simulink model "UAVTrimh"  (R2022a)
settings: Solver=ode45  StartTime=0.0  StopTime=50  RelTol=1e-3  EnableMultiTasking=on
values from neighbouring files (symbols this model uses):
  W = 2.5    [Calculos00_OriginalIgnacio.m]    (also in Calculos02_Vnoladetrim.m; Calculos03_TablaTrimados.m; GenerateDataset_v0.m; PI_0_OnlyOneController_V20.m)
  XCG = 0.33    [Calculos00_OriginalIgnacio.m]    (also in Calculos02_Vnoladetrim.m; Calculos03_TablaTrimados.m; GenerateDataset_v0.m; PI_0_OnlyOneController_V20.m)
settings Model: Creator=Ignacio  LastModifiedBy=ignac
settings SolverCC: AlgebraicLoopSolver=TrustRegion
settings DataIOCC: ExternalInput=[0 0.369809473744665 -0.0760167506859634 0.299999999999976]  InitialState=[]  LimitDataPoints=on  SaveFormat=Array  SignalLoggingSaveFormat=ModelDataLogs  ReturnWorkspaceOutputs=off
settings OptimizationCC: DefaultParameterBehavior=Inlined  BufferReuse=off  ExpressionDepthLimit=2147483647  LifeSpan=inf
settings DebuggingCC: UnderspecifiedInitializationDetection=Classic  MergeDetectMultiDrivingBlocksExec=none  FcnCallInpInsideContextMsg=warning  UnconnectedInputMsg=warning  UnconnectedOutputMsg=warning  UnconnectedLineMsg=warning  StateNameClashWarn=warning  InitInArrayFormatMsg=none  SFUnexpectedBacktrackingDiag=warning  SFNoUnconditionalDefaultTransitionDiag=warning  SFExecutionAtInitializationDiag=none  SFMachineParentedDataDiag=warning  ArithmeticOperatorsInVariantConditions=warning
settings HardwareCC: ProdBitPerPointer=32  ProdBitPerSizeT=32  ProdBitPerPtrDiffT=32  ProdLargestAtomicFloat=None  ProdIntDivRoundTo=Undefined  ProdEndianess=Unspecified  ProdWordSize=32  ProdHWDeviceType=32-bit Generic
settings ModelReferenceCC: PropagateSignalLabelsOutOfModel=off
settings SFSimCC: SimUseLocalCustomCode=off  CustomCodeUndefinedFunction=UseInterfaceOnly
settings RTWCC: RTWUseLocalCustomCode=off
settings CodeAppCC: StateflowObjectComments=on
settings GRTTargetCC: TargetLangStandard=C89/C90 (ANSI)
settings ConfigComp: CovMetricSettings=dw  CovSaveCumulativeToWorkspaceVar=on  CovSaveSingleToWorkspaceVar=on  CovExternalEMLEnable=off

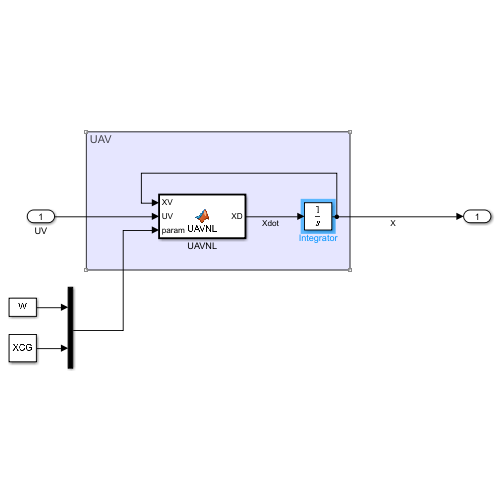
[thumbnail: Simulink's stored preview of the top-level diagram]
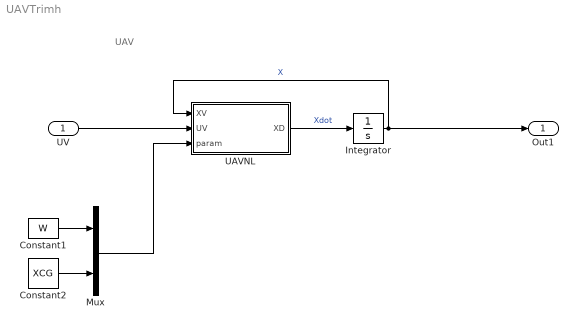
== system UAVTrimh ==
  note: UAV
  UV : Inport  PortDimensions=2
  Constant1 : Constant  Value=W
  Constant2 : Constant  Value=XCG
  Integrator : Integrator  InitialCondition=zeros(1,5)
  Mux : Mux  Inputs=2
  UAVNL : MATLAB Function  TreatAsAtomicUnit=on
  Out1 : Outport
  wires:
  UAVNL/1(XD) -> Integrator/1  "Xdot"
  Integrator/1 -> Out1/1, UAVNL/1(XV)  "X"
  UV/1 -> UAVNL/2(UV)
  Constant1/1 -> Mux/1
  Constant2/1 -> Mux/2
  Mux/1 -> UAVNL/3(param)

== matlab function UAVTrimh/UAVNL ==
  data: XV input; XD output; UV input; param input
function XD = UAVNL(XV,UV,param)

XD=zeros(5,1); % Inicializamos el vector de las derivadas con ceros

% DATOS DE LA AERONAVE

S = 0.4121;               % superficie alar (m^2)
C=0.2192;                  % cuerda media aerodinámica (m)
MASA=2.5;                  % Masa (Kg)
XCGR=0.33;                % posición de referencia del CG
IP=0.156794;                   % Momento de inercia (Kg*m^2)
d=1.225;                      % densidad (Kg/m^3)
G=9.8;                    % gravedad m/s^2
XCG=.33;                  % CG no coincide con el de referencia

% derivadas de estabilidad y control adimensionales

CLalpha0=0.405;    
CLalpha=5.379292;
CLq=11.133615;
CD0=0.0277;
CDalpha=0.14897;
CDalpha2=0.9848;
Cm0=0.0418;     
Cmalpha=-6.0; %1.812981 Más inestable en cabeceo
Cmalphadot=-7.0;
Cmde=-1.552;
Cmq=-18.422237;

% variables de estado


VT=XV(1);	% Velocidad 
ALPHA=XV(2);	% Angulo de ataque
THETA=XV(3);% Angulo de asiento
Q=XV(4);	% Velocidad angular de cabeceo
H=XV(5);

% variables de control

Dt=UV(1);	% Acelerador
De=UV(2);	% Deflexión del timón de profundidad

% parameters

MASA=param(1);
XCG=param(2);

% Density at altitude H
d=density(H);

% Algunos calculos previos

U=VT*cos(ALPHA);	% Componentes de la velocidad en ejes cuerpo
W=VT*sin(ALPHA);	

PDS=0.5*d*(VT^2)*S;	% Presión dinámica*Superficie alar

% Parametros Grupo Motopropulsor

Dh=0.254;   % Diametro de la helice (m)

REVmax=222; % Revoluciones maximas del motor (rev/s)

CT0=0.13805; % Coeficientes de traccion
CTj=-0.2049;
REV=REVmax*Dt; % Motor instantaneo
J=VT/(REV*Dh);  %Coef de velocidad
C_T=CT0+CTj*J;          %Coef de traccion
T=C_T*d*REV^2*Dh^4;     %Traccion

% coeficientes adimensionales de fuerzas y momentos (ejes viento)

CLT=CLalpha0+CLalpha*ALPHA+CLq*Q*C*0.5/VT;         
CDT=CD0+CDalpha*ALPHA+CDalpha2*ALPHA^2;  
CZ=-CDT*sin(ALPHA)-CLT*cos(ALPHA); % Cz en ejes cuerpo para añadir despues el efecto del centro de gravedad
CmT=Cm0+(Cmalpha*ALPHA)+(Cmde*De)+(CZ*(XCG-XCGR))+(C*0.5*Cmq*Q/VT); % Falta la componente alphadot,la añadiremos despues

% Fuerzas aerodinámicas

L=CLT*PDS;
D=CDT*PDS;

% Sistema de ecuaciones diferenciales de la dinámica del vuelo


UDOT=-Q*W+(T-MASA*G*sin(THETA)-D*cos(ALPHA)+L*sin(ALPHA))/MASA;
WDOT=Q*U+(MASA*G*cos(THETA)-D*sin(ALPHA)-L*cos(ALPHA))/MASA;
ALPHADOT=((U*WDOT-W*UDOT)/VT^2);
CmT=CmT+Cmalphadot*C/(2*VT)*ALPHADOT; % Completamos Cm
QDOT=CmT*PDS*C/IP;

VTDOT=(U*UDOT+W*WDOT)/VT;

% Construimos el vector con las derivadas de las variables de estado


XD(1)=VTDOT;
XD(2)=ALPHADOT;
XD(3)=Q;
XD(4)=QDOT;
XD(5)=VT*sin(THETA-ALPHA);
